simulink model "STANDALONE_nav420_Nav_Mode"  (Simulink 7.4)
settings: Solver=ode3  StartTime=0.0  StopTime=inf  RelTol=1e-3
undefined symbols (not defined in the file or in its folder): serial
libraries: instrumentlib x3, NAV420Lib x2, NAV420DecodeLib x1
settings Model: Creator=djulzz  LastModifiedBy=djulzz
settings DebuggingCC: SolverPrmCheckMsg=none

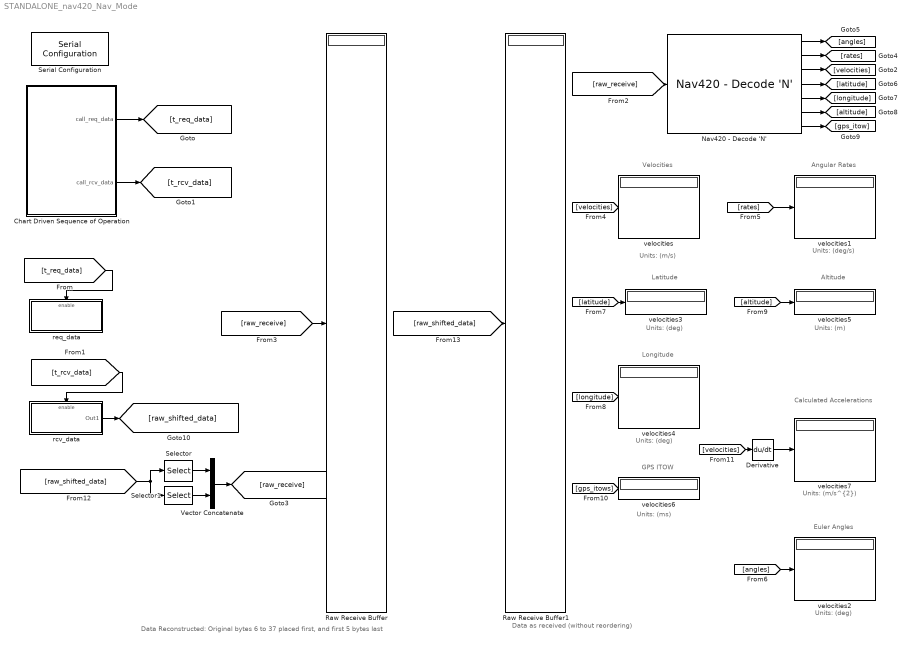
== system STANDALONE_nav420_Nav_Mode ==
  note: Velocities
  note: Units: (m/s)
  note: Angular Rates
  note: Units: (deg/s)
  note: Euler Angles
  note: Units: (deg)
  note: Latitude
  note: Units: (deg)
  note: Longitude
  note: Units: (deg)
  note: Altitude
  note: Units: (m)
  note: GPS ITOW
  note: Units: (ms)
  note: Calculated
      |  Accelerations
  note: Units: (m/s^{2})
  note: Data Reconstructed: Original bytes 6 to 37 placed first,
      |  and first 5 bytes last
  note: Data as received (without reordering)
  Chart Driven Sequence of Operation : Stateflow chart
  Derivative : Derivative
  Nav420 - Decode 'N' : NAV420DecodeLib/Nav420 - Decode 'N'  SystemSampleTime=-1
  Raw Receive Buffer : Display
      settings: Format=hex (Stored Integer)
  Raw Receive Buffer1 : Display
      settings: Format=hex (Stored Integer)
  Selector : Selector  InputPortWidth=37  IndexOptions=Index vector (dialog)  Indices=[6 7 8 9 10 11 12 13 14 15 16 17 18 19 20 21 22 23 24 25 26 27 28 29 30 31 32 33 34 35 36 37]  OutputSizes=1
  Selector1 : Selector  InputPortWidth=37  IndexOptions=Index vector (dialog)  Indices=[1 2 3 4 5]  OutputSizes=1
  Serial Configuration : instrumentlib/Serial Configuration  Priority=-200000  DialogController=instrumentcreatedialog  DialogControllerArgs=DataTag0  ComPortMenu=COM1  ComPort=COM1  ObjConstructor=serial('COM1');  BaudRate=38400  DataBits=8  Parity=none  StopBits=1  FlowControl=none  Timeout=10  ByteOrder=LittleEndian
  Vector Concatenate : Concatenate  Mode=Vector
  rcv_data : Subsystem  TreatAsAtomicUnit=on
  req_data : Subsystem  TreatAsAtomicUnit=on
  velocities{,1..7} (8 alike) : Display
  wires:
  Chart Driven Sequence of Operation/1(call_req_data) -> [t_req_data]
  Chart Driven Sequence of Operation/2(call_rcv_data) -> [t_rcv_data]
  [raw_receive] -> Raw Receive Buffer/1
  [t_req_data] -> req_data/Enable
  [t_rcv_data] -> rcv_data/Enable
  Nav420 - Decode 'N'/3 -> [velocities]
  Selector/1 -> Vector Concatenate/1
  Selector1/1 -> Vector Concatenate/2
  [velocities] -> velocities/1
  rcv_data/1(Out1) -> [raw_shifted_data]
  Vector Concatenate/1 -> [raw_receive]
  [raw_receive] -> Nav420 - Decode 'N'/1
  Nav420 - Decode 'N'/1 -> [angles]
  Nav420 - Decode 'N'/2 -> [rates]
  Nav420 - Decode 'N'/4 -> [latitude]
  Nav420 - Decode 'N'/5 -> [longitude]
  Nav420 - Decode 'N'/6 -> [altitude]
  Nav420 - Decode 'N'/7 -> [gps_itow]
  [rates] -> velocities1/1
  [angles] -> velocities2/1
  [latitude] -> velocities3/1
  [longitude] -> velocities4/1
  [altitude] -> velocities5/1
  [gps_itows] -> velocities6/1
  [velocities] -> Derivative/1
  Derivative/1 -> velocities7/1
  [raw_shifted_data] -> Selector/1, Selector1/1
  [raw_shifted_data] -> Raw Receive Buffer1/1

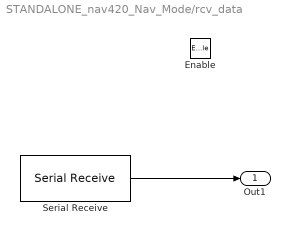
== system STANDALONE_nav420_Nav_Mode/rcv_data ==
  Enable : EnablePort
  Serial Receive : instrumentlib/Serial Receive  DialogController=instrumentcreatedialog  DialogControllerArgs=DataTag1  ComPortMenu=COM1  ComPort=COM1  ObjConstructor=serial('COM1');  Terminator=<none>  DataSize="[37   1]"  DataType=uint8  EnableBlockingMode=on  ActionDataUnavailable=Output last received value  CustomValue=0  SampleTime=-1
  Out1 : Outport  DataType=uint8  OutDataType=fixdt(1, 16)  OutScaling=2^0  OutDataTypeStr=uint8
  wires:
  Serial Receive/1 -> Out1/1

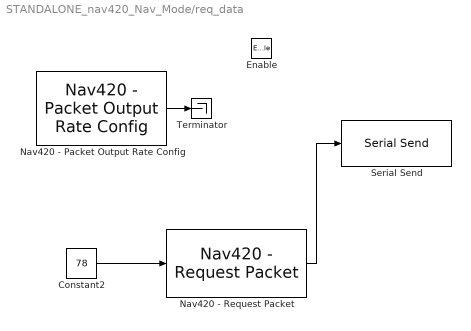
== system STANDALONE_nav420_Nav_Mode/req_data ==
  Enable : EnablePort
  Constant2 : Constant  Value=78  OutDataTypeMode=int8  OutDataType=fixdt(1, 16)  OutScaling=2^0  OutDataTypeStr=int8  SampleTime=-1
  Nav420 - Packet Output Rate Config : NAV420Lib/Nav420 - Packet Output Rate Config  SystemSampleTime=-1  shouldSave=on  output_rate=0
  Nav420 - Request Packet : NAV420Lib/Nav420 - Request Packet  SystemSampleTime=-1
  Serial Send : instrumentlib/Serial Send  DialogController=instrumentcreatedialog  DialogControllerArgs=DataTag2  ComPortMenu=COM1  ComPort=COM1  ObjConstructor=serial('COM1');  Terminator=<none>  EnableBlockingMode=on
  Terminator : Terminator
  wires:
  Constant2/1 -> Nav420 - Request Packet/1
  Nav420 - Packet Output Rate Config/1 -> Terminator/1
  Nav420 - Request Packet/1 -> Serial Send/1

== stateflow chart Chart Driven Sequence of Operation ==
  state Step1
    call_req_data=1;
  state Step2
    call_req_data=0;
  state Step3
    call_rcv_data=1;
  state Step4
    call_rcv_data=0;
  (default) -> Step1
  Step1 -> Step2
  Step2 -> Step3
  Step3 -> Step4
  Step4 -> Step1
  data: call_req_data output uint8; call_rcv_data output uint8
